simulink model "NonLinearHeliInteger"  (R2021a)
settings: Solver=VariableStepAuto  StartTime=0.0  StopTime=10.0  MaxStep=1e-3  RelTol=1e-3
values from neighbouring files (symbols this model uses):
  A = [0 0 1 0 ... (first row only)    [HeliControlGain.m]    (also in HeliControlHinf.m; HeliControlInteger.m; HeliControlLQG.m; HeliControlLQRgain.m)
  B = [0 0 ... (first row only)    [HeliControlGain.m]    (also in HeliControlHinf.m; HeliControlInteger.m; HeliControlLQG.m; HeliControlLQRgain.m)
  Bp = 0.8    [HeliControlGain.m]    (also in HeliControlHinf.m; HeliControlInteger.m; HeliControlIntegerObsv.m; HeliControlLQG.m)
  By = 0.318    [HeliControlGain.m]    (also in HeliControlHinf.m; HeliControlInteger.m; HeliControlIntegerObsv.m; HeliControlLQG.m)
  C = [1 0 0 0 ... (first row only)    [HeliControlGain.m]    (also in HeliControlHinf.m; HeliControlInteger.m; HeliControlLQG.m; HeliControlLQRgain.m)
  g = 9.81    [HeliControlGain.m]    (also in HeliControlHinf.m; HeliControlInteger.m; HeliControlIntegerObsv.m; HeliControlLQG.m)
  Jeq_y = 0.0432    [HeliControlGain.m]    (also in HeliControlHinf.m; HeliControlInteger.m; HeliControlIntegerObsv.m; HeliControlLQG.m)
  Jtp = Jeq_p + Mheli*Lcm^2    (= 0.0863915712)    [HeliControlGain.m]    (also in HeliControlHinf.m; HeliControlInteger.m; HeliControlIntegerObsv.m; HeliControlLQG.m)
  Kf = K(:,1:4)    [HeliControlInteger.m]    (also in HeliControlIntegerObsv.m; HeliControlLQG.m; HeliControlLQRinteger.m)
  Ki = K(:,5:end)    [HeliControlInteger.m]    (also in HeliControlIntegerObsv.m; HeliControlLQG.m; HeliControlLQRinteger.m)
  Kpp = 0.204    [HeliControlGain.m]    (also in HeliControlHinf.m; HeliControlInteger.m; HeliControlIntegerObsv.m; HeliControlLQG.m)
  Kpy = 0.0068    [HeliControlGain.m]    (also in HeliControlHinf.m; HeliControlInteger.m; HeliControlIntegerObsv.m; HeliControlLQG.m)
  Kyp = 0.0219    [HeliControlGain.m]    (also in HeliControlHinf.m; HeliControlInteger.m; HeliControlIntegerObsv.m; HeliControlLQG.m)
  Kyy = 0.072    [HeliControlGain.m]    (also in HeliControlHinf.m; HeliControlInteger.m; HeliControlIntegerObsv.m; HeliControlLQG.m)
  Lcm = 0.186    [HeliControlGain.m]    (also in HeliControlHinf.m; HeliControlInteger.m; HeliControlIntegerObsv.m; HeliControlLQG.m)
  Mheli = 1.3872    [HeliControlGain.m]    (also in HeliControlHinf.m; HeliControlInteger.m; HeliControlIntegerObsv.m; HeliControlLQG.m)
  u0 = a\b    [HeliControlGain.m]    (also in HeliControlHinf.m; HeliControlInteger.m; HeliControlIntegerObsv.m; HeliControlLQG.m)
libraries: simulink x6
settings Model: Creator=Ciro  LastModifiedBy=Ciro

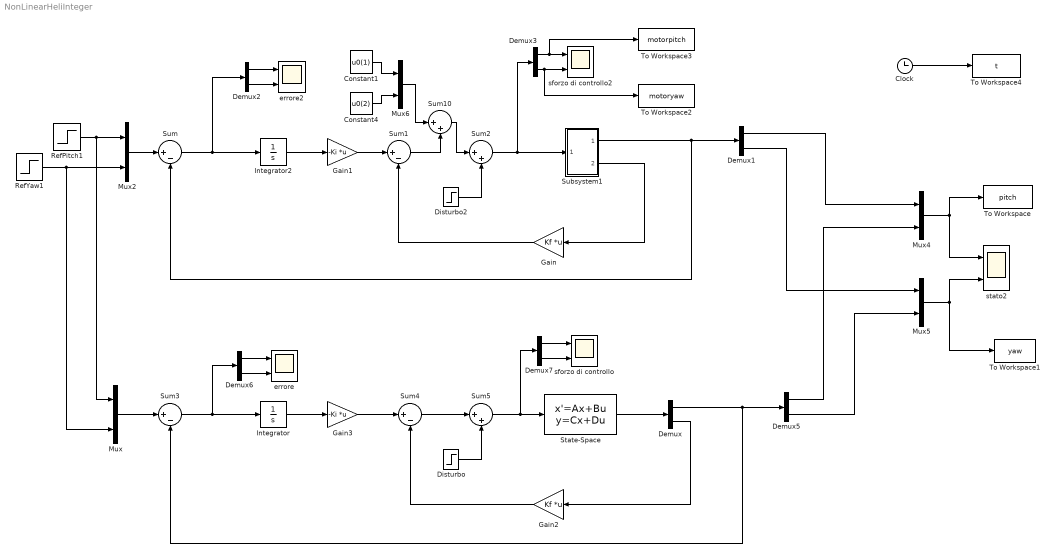
== system NonLinearHeliInteger ==
  Clock : Clock
  Constant1 : Constant  Value=u0(1)
  Constant4 : Constant  Value=u0(2)
  Demux : Demux  Outputs=[2 4]
  Demux{1..3,5..7} (6 alike) : Demux  Outputs=2
  Disturbo : Step  Time=7  After=0.5  SampleTime=0
  Disturbo2 : Step  Time=7  After=0.5  SampleTime=0
  Gain : Gain  Gain=Kf  Multiplication=Matrix(K*u)
  Gain1 : Gain  Gain=-Ki  Multiplication=Matrix(K*u)
  Gain2 : Gain  Gain=Kf  Multiplication=Matrix(K*u)
  Gain3 : Gain  Gain=-Ki  Multiplication=Matrix(K*u)
  Integrator : Integrator
  Integrator2 : Integrator
  Mux{,2,4..6} (5 alike) : Mux  Inputs=2
  RefPitch1 : Step  After=0.3  SampleTime=0
  RefYaw1 : Step  After=0.3  SampleTime=0
  State-Space : StateSpace  A=A  B=B  C=[C; eye(4)]  D=zeros(6,2)  InitialCondition=0
  Subsystem1 : Subsystem
  Sum{,1,3..4} (4 alike) : Sum  Inputs=|+-
  Sum10 : Sum  Inputs=|++
  Sum2 : Sum  Inputs=|++
  Sum5 : Sum  Inputs=|++
  To Workspace : ToWorkspace  VariableName=pitch  SampleTime=-1
      settings: Save2DSignal=2-D array (concatenate along first dimension)
  To Workspace1 : ToWorkspace  VariableName=yaw  SampleTime=-1
      settings: Save2DSignal=2-D array (concatenate along first dimension)
  To Workspace2 : ToWorkspace  VariableName=motoryaw  SampleTime=-1
      settings: Save2DSignal=2-D array (concatenate along first dimension)
  To Workspace3 : ToWorkspace  VariableName=motorpitch  SampleTime=-1
      settings: Save2DSignal=2-D array (concatenate along first dimension)
  To Workspace4 : ToWorkspace  VariableName=t  SampleTime=-1
      settings: Save2DSignal=2-D array (concatenate along first dimension)
  errore : Scope  NumInputPorts=2
  errore2 : Scope  NumInputPorts=2
  sforzo di controllo : Scope  NumInputPorts=2
  sforzo di controllo2 : Scope  NumInputPorts=2
  stato2 : Scope  NumInputPorts=2
  wires:
  Subsystem1/2(Out2) -> Gain/1
  RefPitch1/1 -> Mux/1, Mux2/1
  Demux3/2 -> sforzo di controllo2/2, To Workspace2/1
  Demux3/1 -> To Workspace3/1, sforzo di controllo2/1
  Demux2/2 -> errore2/2
  Disturbo2/1 -> Sum2/2
  Demux1/1 -> Mux4/1
  Demux2/1 -> errore2/1
  Demux1/2 -> Mux5/1
  RefYaw1/1 -> Mux/2, Mux2/2
  Sum2/1 -> Demux3/1, Subsystem1/1(In1)
  Mux2/1 -> Sum/1
  Integrator2/1 -> Gain1/1
  Gain/1 -> Sum1/2
  Sum/1 -> Demux2/1, Integrator2/1
  Gain1/1 -> Sum1/1
  Mux6/1 -> Sum10/1
  Constant1/1 -> Mux6/1
  Constant4/1 -> Mux6/2
  Sum1/1 -> Sum10/2
  Sum10/1 -> Sum2/1
  Demux7/2 -> sforzo di controllo/2
  Demux7/1 -> sforzo di controllo/1
  Demux6/2 -> errore/2
  Disturbo/1 -> Sum5/2
  Sum4/1 -> Sum5/1
  Demux5/1 -> Mux4/2
  Demux6/1 -> errore/1
  Demux5/2 -> Mux5/2
  Sum5/1 -> Demux7/1, State-Space/1
  Mux/1 -> Sum3/1
  Integrator/1 -> Gain3/1
  Gain2/1 -> Sum4/2
  Sum3/1 -> Demux6/1, Integrator/1
  Gain3/1 -> Sum4/1
  Mux4/1 -> stato2/1, To Workspace/1
  Mux5/1 -> To Workspace1/1, stato2/2
  State-Space/1 -> Demux/1
  Demux/1 -> Demux5/1, Sum3/2
  Demux/2 -> Gain2/1
  Subsystem1/1(Out1) -> Demux1/1, Sum/2
  Clock/1 -> To Workspace4/1

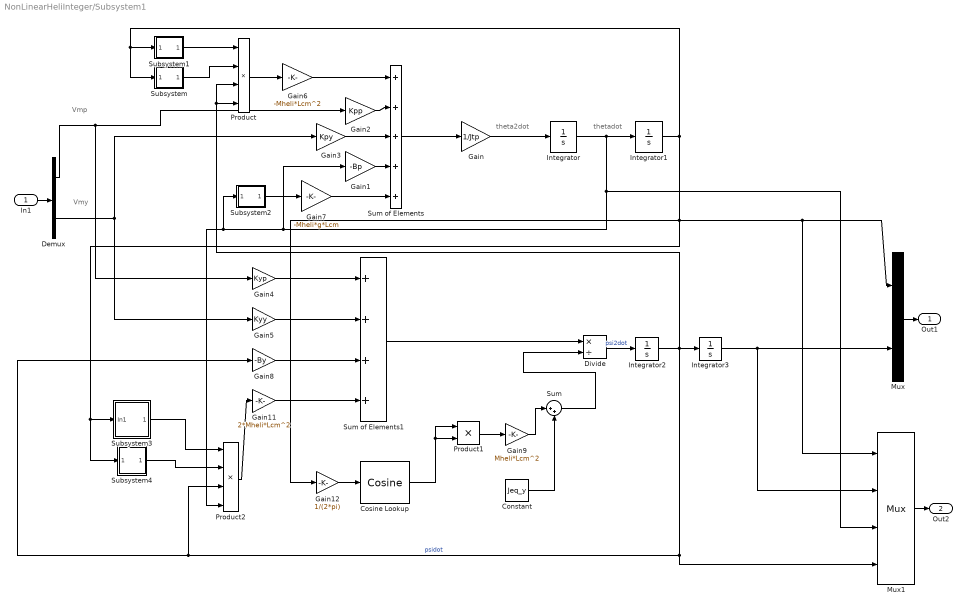
== system NonLinearHeliInteger/Subsystem1 ==
  note: Vmp
  note: Vmy
  note: thetadot
  note: theta2dot
  In1 : Inport
  Constant : Constant  Value=Jeq_y
  Cosine Lookup : simulink/Lookup Tables/Cosine  Formula=cos(2*pi*u)  NumDataPoints=(2^5)+1  OutputWordLength=16  InternalRulePriority=Speed
      settings: SourceProductBaseCode=SL
  Demux : Demux  Outputs=2
  Divide : Product  Inputs=*/
  Gain : Gain  Gain=1/Jtp
  Gain1 : Gain  Gain=-Bp
  Gain11 : Gain  Gain=2*Mheli*Lcm^2
  Gain12 : Gain  Gain=1/(2*pi)
  Gain2 : Gain  Gain=Kpp
  Gain3 : Gain  Gain=Kpy
  Gain4 : Gain  Gain=Kyp
  Gain5 : Gain  Gain=Kyy
  Gain6 : Gain  Gain=-Mheli*Lcm^2
  Gain7 : Gain  Gain=-Mheli*g*Lcm
  Gain8 : Gain  Gain=-By
  Gain9 : Gain  Gain=Mheli*Lcm^2
  Integrator{,1..3} (4 alike) : Integrator
  Mux : Mux  Inputs=2
  Mux1 : Mux
  Product : Product  Inputs=4
  Product1 : Product
  Product2 : Product  Inputs=4
  Subsystem : Subsystem
  Subsystem1 : Subsystem
  Subsystem2 : Subsystem
  Subsystem3 : Subsystem
  Subsystem4 : Subsystem
  Sum : Sum  Inputs=|++
  Sum of Elements : Sum  Inputs=+++++
  Sum of Elements1 : Sum  Inputs=++++
  Out1 : Outport
  Out2 : Outport  Port=2
  wires:
  Subsystem3/1(cos(2*pi*u)) -> Product2/1
  Integrator/1 -> Mux1/3, Gain1/1, Product2/4, Subsystem2/1(In1), Integrator1/1
  Product2/1 -> Gain11/1
  Integrator1/1 -> Subsystem4/1(In1), Subsystem3/1(In1), Mux1/1, Mux/1, Gain12/1, Subsystem/1(In1), Subsystem1/1(In1)
  Gain1/1 -> Sum of Elements/4
  Sum of Elements/1 -> Gain/1
  Sum/1 -> Divide/2
  Gain/1 -> Integrator/1
  Integrator2/1 -> Product/4, Product/3, Mux1/4, Gain8/1, Product2/3, Integrator3/1  "psidot"
  Subsystem2/1(cos(2*pi*u)) -> Gain7/1
  Demux/2 -> Gain5/1, Gain3/1
  Demux/1 -> Gain4/1, Gain2/1
  Integrator3/1 -> Mux1/2, Mux/2
  Gain7/1 -> Sum of Elements/5
  Product/1 -> Gain6/1
  Gain8/1 -> Sum of Elements1/3
  Gain4/1 -> Sum of Elements1/1
  Mux/1 -> Out1/1
  Gain11/1 -> Sum of Elements1/4
  Divide/1 -> Integrator2/1  "psi2dot"
  Cosine Lookup/1 -> Product1/2, Product1/1
  Sum of Elements1/1 -> Divide/1
  Gain2/1 -> Sum of Elements/2
  Gain12/1 -> Cosine Lookup/1
  Mux1/1 -> Out2/1
  Subsystem4/1(sin(2*pi*u)) -> Product2/2
  Constant/1 -> Sum/2
  Subsystem/1(cos(2*pi*u)) -> Product/2
  Gain6/1 -> Sum of Elements/1
  Gain3/1 -> Sum of Elements/3
  Subsystem1/1(sin(2*pi*u)) -> Product/1
  Product1/1 -> Gain9/1
  In1/1 -> Demux/1
  Gain9/1 -> Sum/1
  Gain5/1 -> Sum of Elements1/2

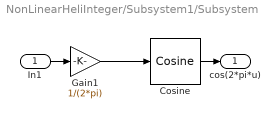
== system NonLinearHeliInteger/Subsystem1/Subsystem ==
  In1 : Inport
  Cosine : simulink/Lookup Tables/Cosine  Formula=cos(2*pi*u)  NumDataPoints=(2^5)+1  OutputWordLength=16  InternalRulePriority=Speed
      settings: SourceProductBaseCode=SL
  Gain1 : Gain  Gain=1/(2*pi)
  cos(2*pi*u) : Outport
  wires:
  Gain1/1 -> Cosine/1
  In1/1 -> Gain1/1
  Cosine/1 -> cos(2*pi*u)/1

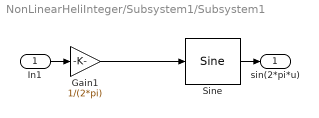
== system NonLinearHeliInteger/Subsystem1/Subsystem1 ==
  In1 : Inport
  Gain1 : Gain  Gain=1/(2*pi)
  Sine : simulink/Lookup Tables/Sine  Formula=sin(2*pi*u)  NumDataPoints=(2^5)+1  OutputWordLength=16  InternalRulePriority=Speed
  sin(2*pi*u) : Outport
  wires:
  Gain1/1 -> Sine/1
  In1/1 -> Gain1/1
  Sine/1 -> sin(2*pi*u)/1

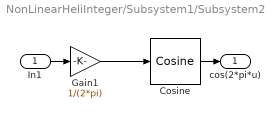
== system NonLinearHeliInteger/Subsystem1/Subsystem2 ==
  In1 : Inport
  Cosine : simulink/Lookup Tables/Cosine  Formula=cos(2*pi*u)  NumDataPoints=(2^5)+1  OutputWordLength=16  InternalRulePriority=Speed
      settings: SourceProductBaseCode=SL
  Gain1 : Gain  Gain=1/(2*pi)
  cos(2*pi*u) : Outport
  wires:
  Cosine/1 -> cos(2*pi*u)/1
  In1/1 -> Gain1/1
  Gain1/1 -> Cosine/1

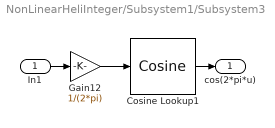
== system NonLinearHeliInteger/Subsystem1/Subsystem3 ==
  In1 : Inport
  Cosine Lookup1 : simulink/Lookup Tables/Cosine  Formula=cos(2*pi*u)  NumDataPoints=(2^5)+1  OutputWordLength=16  InternalRulePriority=Speed
      settings: SourceProductBaseCode=SL
  Gain12 : Gain  Gain=1/(2*pi)
  cos(2*pi*u) : Outport
  wires:
  Gain12/1 -> Cosine Lookup1/1
  In1/1 -> Gain12/1
  Cosine Lookup1/1 -> cos(2*pi*u)/1

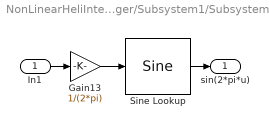
== system NonLinearHeliInteger/Subsystem1/Subsystem4 ==
  In1 : Inport
  Gain13 : Gain  Gain=1/(2*pi)
  Sine Lookup : simulink/Lookup Tables/Sine  Formula=sin(2*pi*u)  NumDataPoints=(2^5)+1  OutputWordLength=16  InternalRulePriority=Speed
  sin(2*pi*u) : Outport
  wires:
  Gain13/1 -> Sine Lookup/1
  Sine Lookup/1 -> sin(2*pi*u)/1
  In1/1 -> Gain13/1
